simulink model "rostest"  (R2021a)
settings: Solver=VariableStepAuto  StartTime=0.0  StopTime=10000  RelTol=1e-3
libraries: robotlib x2
settings Model: Creator=lsh  LastModifiedBy=lsh

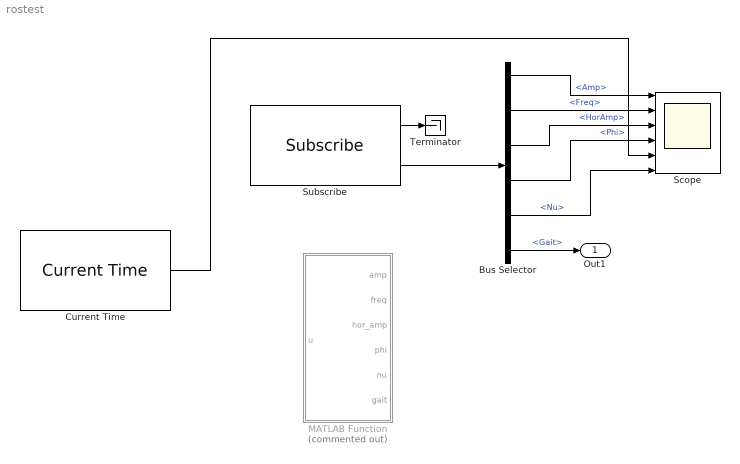
== system rostest ==
  Bus Selector : BusSelector  OutputSignals=Amp,Freq,HorAmp,Phi,Nu,Gait
  Current Time : robotlib/Current Time  OutputFormat=bus  SampleTime=-1  ModelName=robotlib
      settings: SourceProductBaseCode=RR
  MATLAB Function : MATLAB Function  Commented=on  TreatAsAtomicUnit=on
  Scope : Scope  NumInputPorts=6
  Subscribe : robotlib/Subscribe  topicSource=Specify your own  topic=/gait_param  messageType=snake_panel/gaitparam  SampleTime=-1  legacyBusStruct=off  messageQueueLength=1
  Terminator : Terminator
  Out1 : Outport
  wires:
  Subscribe/2 -> Bus Selector/1
  Bus Selector/1 -> Scope/1  "<Amp>"
  Bus Selector/2 -> Scope/2  "<Freq>"
  Bus Selector/3 -> Scope/3  "<HorAmp>"
  Bus Selector/4 -> Scope/4  "<Phi>"
  Bus Selector/5 -> Scope/6  "<Nu>"
  Bus Selector/6 -> Out1/1  "<Gait>"
  Subscribe/1 -> Terminator/1
  Current Time/1 -> Scope/5

== matlab function rostest/MATLAB Function ==
  data: u input; amp output; freq output; hor_amp output; phi output; nu output; gait output
function [amp, freq, hor_amp, phi, nu, gait]= fcn(u)
    sub = rossubscriber('/gait_param', 'snake_panel/gaitparam', @callback);
